simulink model "Exer3_3_2"  (R2014b)
settings: Solver=ode45  StartTime=0.0  StopTime=2  RelTol=1e-3
settings Model: Creator=Charlie  LastModifiedBy=Charlie

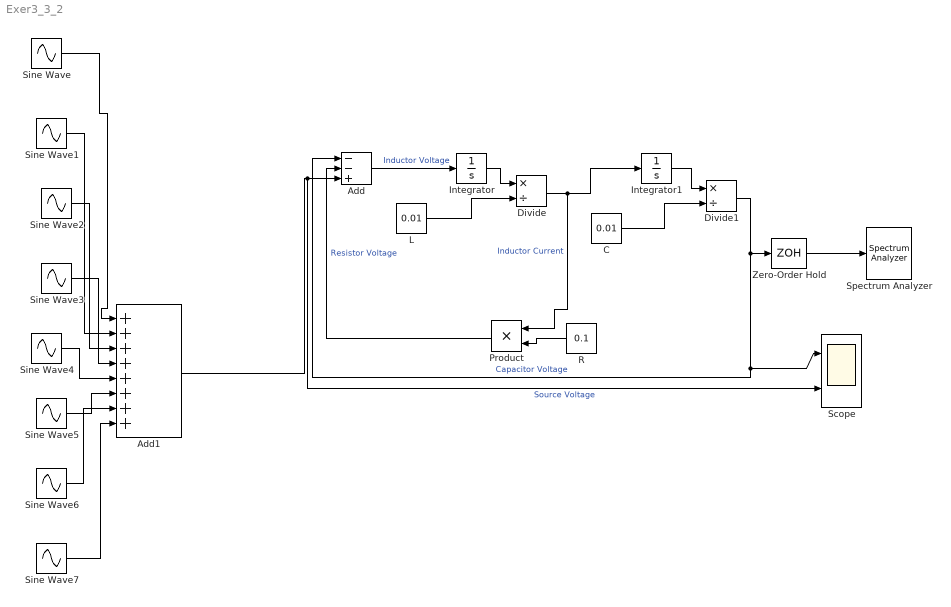
== system Exer3_3_2 ==
  Add : Sum  Inputs=--+
  Add1 : Sum  Inputs=++++++++
  C : Constant  Value=0.01
  Divide : Product  Inputs=*/
  Divide1 : Product  Inputs=*/
  Integrator : Integrator
  Integrator1 : Integrator
  L : Constant  Value=0.01
  Product : Product
  R : Constant  Value=0.1
  Scope : Scope  NumInputPorts=2
      settings: YMin=-2~-1  YMax=2~1
  Sine Wave : Sin  Amplitude=0.112  Frequency=1407.4  SampleTime=0
  Sine Wave1 : Sin  Amplitude=0.7854  Frequency=201.062  SampleTime=0
  Sine Wave2 : Sin  Amplitude=0.262  Frequency=603.2  SampleTime=0
  Sine Wave3 : Sin  Amplitude=0.157  Frequency=1005.3  SampleTime=0
  Sine Wave4 : Sin  Amplitude=0.08727  Frequency=1809.5  SampleTime=0
  Sine Wave5 : Sin  Amplitude=0.0714  Frequency=2211.68  SampleTime=0
  Sine Wave6 : Sin  Amplitude=0.0604  Frequency=2613.8  SampleTime=0
  Sine Wave7 : Sin  Amplitude=0.0524  Frequency=3015.93  SampleTime=0
  Spectrum Analyzer : SpectrumAnalyzer
  Zero-Order Hold : ZeroOrderHold  SampleTime=2e-7
  wires:
  Add/1 -> Integrator/1  "Inductor Voltage"
  Integrator/1 -> Divide/1
  L/1 -> Divide/2
  Divide/1 -> Product/1, Integrator1/1  "Inductor Current"
  Integrator1/1 -> Divide1/1
  C/1 -> Divide1/2
  Divide1/1 -> Zero-Order Hold/1, Add/1, Scope/1  "Capacitor Voltage"
  R/1 -> Product/2
  Product/1 -> Add/2  "Resistor Voltage"
  Zero-Order Hold/1 -> Spectrum Analyzer/1
  Add1/1 -> Add/3, Scope/2  "Source Voltage"
  Sine Wave/1 -> Add1/1
  Sine Wave1/1 -> Add1/2
  Sine Wave2/1 -> Add1/3
  Sine Wave3/1 -> Add1/4
  Sine Wave4/1 -> Add1/5
  Sine Wave5/1 -> Add1/6
  Sine Wave6/1 -> Add1/7
  Sine Wave7/1 -> Add1/8
